simulink model "MCC_impulse"  (R2024a)
settings: Solver=VariableStepAuto  StartTime=0.0  StopTime=80  RelTol=1e-3
model workspace (MAT data in the model file):
  K = 0.45
undefined symbols (not defined in the file): B3
settings Model: Creator=hp  LastModifiedBy=NB
settings SolverCC: AlgebraicLoopSolver=TrustRegion
settings DataIOCC: ReturnWorkspaceOutputs=off
settings DebuggingCC: UnconnectedInputMsg=warning  UnconnectedOutputMsg=warning  UnconnectedLineMsg=warning  ArithmeticOperatorsInVariantConditions=warning
settings ModelReferenceCC: EnableRefExpFcnMdlSchedulingChecks=on
settings SFSimCC: CustomCodeUndefinedFunction=UseInterfaceOnly
settings RTWCC: GPUComputeCapability=3.5

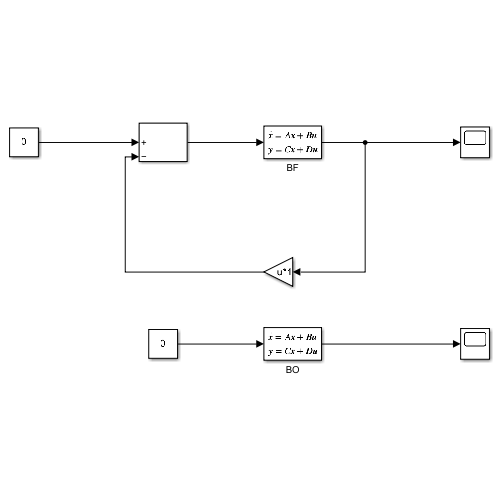
[thumbnail: Simulink's stored preview of the top-level diagram]
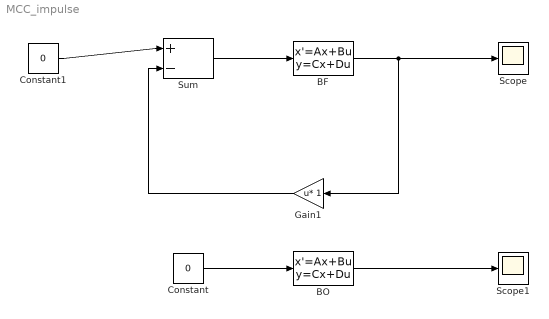
== system MCC_impulse ==
  BF : StateSpace  A=[-2,-0.020000000000000,0;1,-10,0;0,1,0]  B=[2;0;0]  C=[0,0,1]  D=0  InitialCondition=B3
  BO : StateSpace  A=[-2,-0.020000000000000,0;1,-10,0;0,1,0]  B=[2;0;0]  C=[0,0,1]  D=0  InitialCondition=B3
  Constant : Constant  Value=0
  Constant1 : Constant  Value=0
  Gain1 : Gain  Multiplication=Matrix(u*K)
  Scope : Scope
  Scope1 : Scope
  Sum : Sum  Inputs=|+-
  wires:
  Sum/1 -> BF/1
  BF/1 -> Gain1/1, Scope/1
  Gain1/1 -> Sum/2
  Constant/1 -> BO/1
  BO/1 -> Scope1/1
  Constant1/1 -> Sum/1
